simulink model "prob6"  (R2020b)
settings: Solver=FixedStepAuto  StartTime=0.0  StopTime=10.0  RelTol=1e-3
settings Model: Creator=AVM  LastModifiedBy=AVM

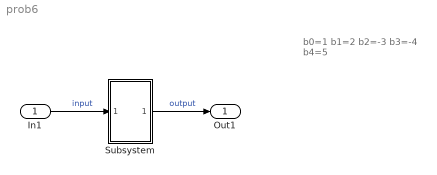
== system prob6 ==
  note: b0=1
      | b1=2
      | b2=-3
      | b3=-4
      | b4=5
  In1 : Inport
  Subsystem : Subsystem
  Out1 : Outport
  wires:
  In1/1 -> Subsystem/1(In1)  "input"
  Subsystem/1(Out1) -> Out1/1  "output"

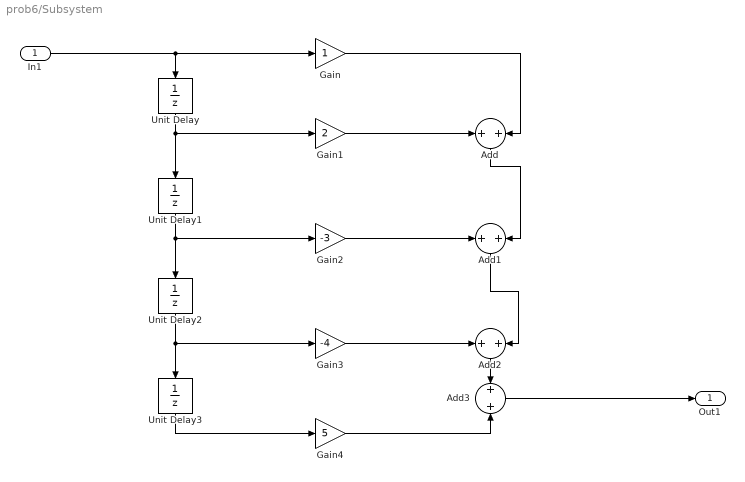
== system prob6/Subsystem ==
  In1 : Inport
  Add{,1..3} (4 alike) : Sum
  Gain : Gain
  Gain1 : Gain  Gain=2
  Gain2 : Gain  Gain=-3
  Gain3 : Gain  Gain=-4
  Gain4 : Gain  Gain=5
  Unit Delay{,1..3} (4 alike) : UnitDelay  SampleTime=-1  HasFrameUpgradeWarning=on
  Out1 : Outport
  wires:
  Unit Delay/1 -> Unit Delay1/1, Gain1/1
  Add/1 -> Add1/2
  Gain4/1 -> Add3/2
  Unit Delay1/1 -> Unit Delay2/1, Gain2/1
  Add1/1 -> Add2/2
  Add2/1 -> Add3/1
  Unit Delay2/1 -> Gain3/1, Unit Delay3/1
  Unit Delay3/1 -> Gain4/1
  Gain1/1 -> Add/1
  Gain/1 -> Add/2
  Gain3/1 -> Add2/1
  Gain2/1 -> Add1/1
  In1/1 -> Unit Delay/1, Gain/1
  Add3/1 -> Out1/1
